simulink model "pi_OfflineRL_H2DF_2023a"  (R2023a)
settings: Solver=FixedStepAuto  StartTime=0.0  StopTime=inf  FixedStep=0.001  RelTol=1e-3  EnableMultiTasking=on
values from neighbouring files (symbols this model uses):
  C2C_NMPC = init_C2C_NMPC_H2DF(C2C_NMPC.expdata)    [init_pi_OfflineRL_H2DF_2023a.m]
  LowerLimit = ([0.17e-3;350;-2;2e-3] - C2C_NMPC.Normalization.controls.mean)./(C2C_NMPC.Normalization.controls.std)    [init_pi_OfflineRL_H2DF_2023a.m]
  UpperLimit = ([0.5e-3;900;10;5.5e-3] - C2C_NMPC.Normalization.controls.mean)./(C2C_NMPC.Normalization.controls.std)    [init_pi_OfflineRL_H2DF_2023a.m]
undefined symbols (not defined in the file or in its folder): DiscIntNeverNeededParam
libraries: deeplib x9, rllib x3, raspberrypiNetworklib x1
(part 1 of 4)
settings Model: VariantConfigurationObject=C2C  SimulationMode=external  ExtModeTrigDuration=2  Creator=maxim  LastModifiedBy=labadmin
settings SolverCC: PositivePriorityOrder=on
settings DataIOCC: LimitDataPoints=on  MaxDataPoints=10000  SaveOutput=off
settings OptimizationCC: EnhancedBackFolding=on  PassReuseOutputArgsAs=Individual arguments  ZeroExternalMemoryAtStartup=off  ZeroInternalMemoryAtStartup=off  MaxStackSize=64  OptimizeBlockOrder=speed  DifferentSizesBufferReuse=on  OptimizationCustomize=off  EfficientTunableParamExpr=on
settings DebuggingCC: ParameterPrecisionLossMsg=none  ParameterTunabilityLossMsg=error
settings HardwareCC: ProdBitPerPointer=32  ProdBitPerSizeT=32  ProdBitPerPtrDiffT=32  ProdLargestAtomicInteger=Long  ProdLargestAtomicFloat=Double  ProdWordSize=32  ProdLongLongMode=on  ProdHWDeviceType=ARM Compatible->ARM Cortex
settings RTWCC: Description=Embedded Coder  SystemTargetFile=ert.tlc  HardwareBoard=Raspberry Pi  TemplateMakefile=ert_default_tmf  RTWUseSimCustomCode=on  Toolchain=GNU GCC Embedded Linux  BuildConfiguration=Faster Runs
settings CodeAppCC: ForceParamTrailComments=on  IgnoreCustomStorageClasses=off  OperatorAnnotations=on  SimulinkDataObjDesc=on  SFDataObjDesc=on  InsertBlockDesc=on
settings ERTTargetCC: SupportContinuousTime=on  SupportNonInlinedSFcns=on  SupportVariableSizeSignals=on  ExtMode=on  ExtModeStaticAlloc=on  ExtModeMaxTrigDuration=1000  ExtModeMexArgs='192.168.140.200' 1 17725

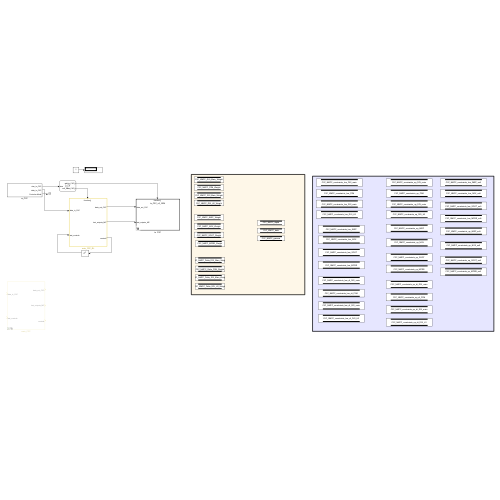
[thumbnail: Simulink's stored preview of the top-level diagram]
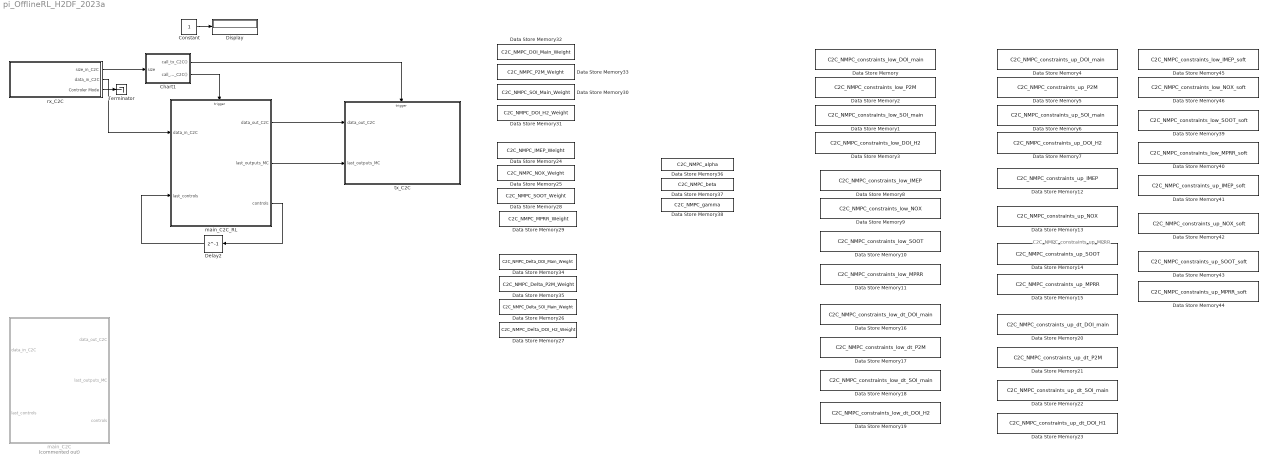
== system pi_OfflineRL_H2DF_2023a ==
  note: C2C_NMPC_constraints_up_MPRR
  Chart1 : Stateflow chart  TreatAsAtomicUnit=on
  Constant : Constant
  Data Store Memory : DataStoreMemory  DataStoreName=C2C_NMPC_constraints_low_DOI_main  WriteAfterWriteMsg=warning  ShowAdditionalParam=off
  Data Store Memory1 : DataStoreMemory  DataStoreName=C2C_NMPC_constraints_low_SOI_main  WriteAfterWriteMsg=warning  ShowAdditionalParam=off
  Data Store Memory10 : DataStoreMemory  DataStoreName=C2C_NMPC_constraints_low_SOOT  WriteAfterWriteMsg=warning  ShowAdditionalParam=off
  Data Store Memory11 : DataStoreMemory  DataStoreName=C2C_NMPC_constraints_low_MPRR  WriteAfterWriteMsg=warning  ShowAdditionalParam=off
  Data Store Memory12 : DataStoreMemory  DataStoreName=C2C_NMPC_constraints_up_IMEP  WriteAfterWriteMsg=warning  ShowAdditionalParam=off
  Data Store Memory13 : DataStoreMemory  DataStoreName=C2C_NMPC_constraints_up_NOX  WriteAfterWriteMsg=warning  ShowAdditionalParam=off
  Data Store Memory14 : DataStoreMemory  DataStoreName=C2C_NMPC_constraints_up_SOOT  WriteAfterWriteMsg=warning  ShowAdditionalParam=off
  Data Store Memory15 : DataStoreMemory  DataStoreName=C2C_NMPC_constraints_up_MPRR  WriteAfterWriteMsg=warning  ShowAdditionalParam=off
  Data Store Memory16 : DataStoreMemory  DataStoreName=C2C_NMPC_constraints_low_dt_DOI_main  WriteAfterWriteMsg=warning  ShowAdditionalParam=off
  Data Store Memory17 : DataStoreMemory  DataStoreName=C2C_NMPC_constraints_low_dt_P2M  WriteAfterWriteMsg=warning  ShowAdditionalParam=off
  Data Store Memory18 : DataStoreMemory  DataStoreName=C2C_NMPC_constraints_low_dt_SOI_main  WriteAfterWriteMsg=warning  ShowAdditionalParam=off
  Data Store Memory19 : DataStoreMemory  DataStoreName=C2C_NMPC_constraints_low_dt_DOI_H2  WriteAfterWriteMsg=warning  ShowAdditionalParam=off
  Data Store Memory2 : DataStoreMemory  DataStoreName=C2C_NMPC_constraints_low_P2M  WriteAfterWriteMsg=warning  ShowAdditionalParam=off
  Data Store Memory20 : DataStoreMemory  DataStoreName=C2C_NMPC_constraints_up_dt_DOI_main  WriteAfterWriteMsg=warning  ShowAdditionalParam=off
  Data Store Memory21 : DataStoreMemory  DataStoreName=C2C_NMPC_constraints_up_dt_P2M  WriteAfterWriteMsg=warning  ShowAdditionalParam=off
  Data Store Memory22 : DataStoreMemory  DataStoreName=C2C_NMPC_constraints_up_dt_SOI_main  WriteAfterWriteMsg=warning  ShowAdditionalParam=off
  Data Store Memory23 : DataStoreMemory  DataStoreName=C2C_NMPC_constraints_up_dt_DOI_H1  WriteAfterWriteMsg=warning  ShowAdditionalParam=off
  Data Store Memory24 : DataStoreMemory  DataStoreName=C2C_NMPC_IMEP_Weight  WriteAfterWriteMsg=warning  ShowAdditionalParam=off
  Data Store Memory25 : DataStoreMemory  DataStoreName=C2C_NMPC_NOX_Weight  WriteAfterWriteMsg=warning  ShowAdditionalParam=off
  Data Store Memory26 : DataStoreMemory  DataStoreName=C2C_NMPC_Delta_SOI_Main_Weight  WriteAfterWriteMsg=warning  ShowAdditionalParam=off
  Data Store Memory27 : DataStoreMemory  DataStoreName=C2C_NMPC_Delta_DOI_H2_Weight  WriteAfterWriteMsg=warning  ShowAdditionalParam=off
  Data Store Memory28 : DataStoreMemory  DataStoreName=C2C_NMPC_SOOT_Weight  WriteAfterWriteMsg=warning  ShowAdditionalParam=off
  Data Store Memory29 : DataStoreMemory  DataStoreName=C2C_NMPC_MPRR_Weight  WriteAfterWriteMsg=warning  ShowAdditionalParam=off
  Data Store Memory3 : DataStoreMemory  DataStoreName=C2C_NMPC_constraints_low_DOI_H2  WriteAfterWriteMsg=warning  ShowAdditionalParam=off
  Data Store Memory30 : DataStoreMemory  DataStoreName=C2C_NMPC_SOI_Main_Weight  WriteAfterWriteMsg=warning  ShowAdditionalParam=off
  Data Store Memory31 : DataStoreMemory  DataStoreName=C2C_NMPC_DOI_H2_Weight  WriteAfterWriteMsg=warning  ShowAdditionalParam=off
  Data Store Memory32 : DataStoreMemory  DataStoreName=C2C_NMPC_DOI_Main_Weight  WriteAfterWriteMsg=warning  ShowAdditionalParam=off
  Data Store Memory33 : DataStoreMemory  DataStoreName=C2C_NMPC_P2M_Weight  WriteAfterWriteMsg=warning  ShowAdditionalParam=off
  Data Store Memory34 : DataStoreMemory  DataStoreName=C2C_NMPC_Delta_DOI_Main_Weight  WriteAfterWriteMsg=warning  ShowAdditionalParam=off
  Data Store Memory35 : DataStoreMemory  DataStoreName=C2C_NMPC_Delta_P2M_Weight  WriteAfterWriteMsg=warning  ShowAdditionalParam=off
  Data Store Memory36 : DataStoreMemory  DataStoreName=C2C_NMPC_alpha  WriteAfterWriteMsg=warning  ShowAdditionalParam=off
  Data Store Memory37 : DataStoreMemory  DataStoreName=C2C_NMPC_beta  WriteAfterWriteMsg=warning  ShowAdditionalParam=off
  Data Store Memory38 : DataStoreMemory  DataStoreName=C2C_NMPC_gamma  WriteAfterWriteMsg=warning  ShowAdditionalParam=off
  Data Store Memory39 : DataStoreMemory  DataStoreName=C2C_NMPC_constraints_low_SOOT_soft  WriteAfterWriteMsg=warning  ShowAdditionalParam=off
  Data Store Memory4 : DataStoreMemory  DataStoreName=C2C_NMPC_constraints_up_DOI_main  WriteAfterWriteMsg=warning  ShowAdditionalParam=off
  Data Store Memory40 : DataStoreMemory  DataStoreName=C2C_NMPC_constraints_low_MPRR_soft  WriteAfterWriteMsg=warning  ShowAdditionalParam=off
  Data Store Memory41 : DataStoreMemory  DataStoreName=C2C_NMPC_constraints_up_IMEP_soft  WriteAfterWriteMsg=warning  ShowAdditionalParam=off
  Data Store Memory42 : DataStoreMemory  DataStoreName=C2C_NMPC_constraints_up_NOX_soft  WriteAfterWriteMsg=warning  ShowAdditionalParam=off
  Data Store Memory43 : DataStoreMemory  DataStoreName=C2C_NMPC_constraints_up_SOOT_soft  WriteAfterWriteMsg=warning  ShowAdditionalParam=off
  Data Store Memory44 : DataStoreMemory  DataStoreName=C2C_NMPC_constraints_up_MPRR_soft  WriteAfterWriteMsg=warning  ShowAdditionalParam=off
  Data Store Memory45 : DataStoreMemory  DataStoreName=C2C_NMPC_constraints_low_IMEP_soft  WriteAfterWriteMsg=warning  ShowAdditionalParam=off
  Data Store Memory46 : DataStoreMemory  DataStoreName=C2C_NMPC_constraints_low_NOX_soft  WriteAfterWriteMsg=warning  ShowAdditionalParam=off
  Data Store Memory5 : DataStoreMemory  DataStoreName=C2C_NMPC_constraints_up_P2M  WriteAfterWriteMsg=warning  ShowAdditionalParam=off
  Data Store Memory6 : DataStoreMemory  DataStoreName=C2C_NMPC_constraints_up_SOI_main  WriteAfterWriteMsg=warning  ShowAdditionalParam=off
  Data Store Memory7 : DataStoreMemory  DataStoreName=C2C_NMPC_constraints_up_DOI_H2  WriteAfterWriteMsg=warning  ShowAdditionalParam=off
  Data Store Memory8 : DataStoreMemory  DataStoreName=C2C_NMPC_constraints_low_IMEP  WriteAfterWriteMsg=warning  ShowAdditionalParam=off
  Data Store Memory9 : DataStoreMemory  DataStoreName=C2C_NMPC_constraints_low_NOX  WriteAfterWriteMsg=warning  ShowAdditionalParam=off
  Delay2 : Delay  DelayLength=1  InitialCondition=C2C_NMPC.x0([(C2C_NMPC.Dims.n_LSTM_states + 1):(C2C_NMPC.Dims.n_LSTM_states + C2C_NMPC.Dims.n_controls)])
  Display : Display
  Terminator : Terminator
  main_C2C : Subsystem  Commented=on  Variant=on  VariantControlMode=label  VariantControl=main_C2C_n3  LabelModeActiveChoice=main_C2C_RL
  main_C2C_RL : Subsystem  VariantControl=main_C2C_RL
  rx_C2C : Subsystem
  tx_C2C : Subsystem  Variant=on  VariantControlMode=label  VariantControl=Choice  LabelModeActiveChoice=tx_C2C_n3_GRU
  wires:
  rx_C2C/1(size_in_C2C) -> Chart1/1(size)
  Chart1/1(call_tx_C2C()) -> tx_C2C/Trigger
  rx_C2C/2(data_in_C2C) -> main_C2C_RL/1(data_in_C2C)
  Delay2/1 -> main_C2C_RL/2(last_controls)
  main_C2C_RL/1(data_out_C2C) -> tx_C2C/1(data_out_C2C)
  main_C2C_RL/3(controls) -> Delay2/1
  main_C2C_RL/2(last_outputs_MC) -> tx_C2C/2(last_outputs_MC)
  Constant/1 -> Display/1
  rx_C2C/3(Controler Mode) -> Terminator/1
  Chart1/2(call_main_C2C()) -> main_C2C_RL/Trigger

== system pi_OfflineRL_H2DF_2023a/main_C2C ==
  note: 192.168.140.200
  data_in_C2C : Inport
  last_controls : Inport  Port=2
  main_C2C_RL : Subsystem  VariantControl=main_C2C_RL
  data_out_C2C : Outport
  last_outputs_MC : Outport  Port=2
  controls : Outport  Port=3

== system pi_OfflineRL_H2DF_2023a/main_C2C_RL ==
  data_in_C2C : Inport
  last_controls : Inport  Port=2
  function : TriggerPort  TriggerType=function-call  VariantControl=(inherit)
  IC : InitialCondition  Value=C2C_NMPC.x0([(C2C_NMPC.Dims.n_LSTM_states + 1):(C2C_NMPC.Dims.n_LSTM_states + C2C_NMPC.Dims.n_controls)])
  RL_Controller : Subsystem  VariantControl=C2C_NMPC_n3
  post_processing : Subsystem
  pre_processing1 : Subsystem
  data_out_C2C : Outport
  last_outputs_MC : Outport  Port=2
  controls : Outport  Port=3
  wires:
  post_processing/1(data_C2C_out) -> data_out_C2C/1
  pre_processing1/2(counter_C2C) -> [counter_C2C]
  [counter_C2C] -> post_processing/5(counter)
  last_controls/1 -> [last_controls]
  RL_Controller/1(status_C2C) -> post_processing/3(controller_status)
  [last_outputs_MC] -> post_processing/4(last_outputs_MC)
  [last_outputs_MC] -> last_outputs_MC/1
  pre_processing1/3(last_outputs_MC) -> RL_Controller/2(last_outputs), [last_outputs_MC]
  data_in_C2C/1 -> pre_processing1/1(data_in_C2C)
  pre_processing1/1(reference_C2C) -> post_processing/1(reference), RL_Controller/1(reference_C2C)
  IC/1 -> controls/1, post_processing/2(controls)
  RL_Controller/3(LSTM_states) -> post_processing/6(LSTM_States)
  RL_Controller/2(controls) -> IC/1

== system pi_OfflineRL_H2DF_2023a/rx_C2C ==
  Data Type Conversion : DataTypeConversion  OutDataTypeStr=double  SaturateOnIntegerOverflow=off  RndMeth=Floor
  Receive : Subsystem
  Subsystem1 : Subsystem  Commented=on
  Subsystem4 : Subsystem  Commented=on
  UDP Receive1 : raspberrypiNetworklib/UDP Receive  localURL='0.0.0.0'  localPort=42785  remoteURL='0.0.0.0'  remotePort=-1  recvBufferSize=8192  signalDatatype=uint32  dims=56  isVarSize=off  showBlockingTime=off  blockingTime=0  sampletime=0.001  blockPlatform=Raspberry Pi
  size_in_C2C : Outport
  data_in_C2C : Outport  Port=2
  Controler Mode : Outport  Port=3
  wires:
  UDP Receive1/2 -> size_in_C2C/1
  UDP Receive1/1 -> Data Type Conversion/1
  Receive/1(udp_outputs) -> data_in_C2C/1
  Data Type Conversion/1 -> Receive/1(udp_data_in)
  Receive/2(controller_mode) -> Controler Mode/1

== system pi_OfflineRL_H2DF_2023a/tx_C2C ==
  data_out_C2C : Inport
  last_outputs_MC : Inport  Port=2
  function : TriggerPort  TriggerType=function-call  VariantControl=(inherit)
  tx_C2C_n3 : Subsystem  VariantControl=tx_C2C_n3
  tx_C2C_n3_GRU : Subsystem  VariantControl=tx_C2C_n3_GRU

== system pi_OfflineRL_H2DF_2023a/main_C2C/main_C2C_RL ==
  data_in_C2C : Inport
  last_controls : Inport  Port=2
  IC : InitialCondition  Value=C2C_NMPC.x0([(C2C_NMPC.Dims.n_LSTM_states + 1):(C2C_NMPC.Dims.n_LSTM_states + C2C_NMPC.Dims.n_controls)])
  RL_Controller : Subsystem  VariantControl=C2C_NMPC_n3
  post_processing : Subsystem
  pre_processing1 : Subsystem
  data_out_C2C : Outport
  last_outputs_MC : Outport  Port=2
  controls : Outport  Port=3
  wires:
  post_processing/1(data_C2C_out) -> data_out_C2C/1
  pre_processing1/2(counter_C2C) -> [counter_C2C]
  [counter_C2C] -> post_processing/5(counter)
  last_controls/1 -> [last_controls]
  RL_Controller/1(status_C2C) -> post_processing/3(controller_status)
  [last_outputs_MC] -> post_processing/4(last_outputs_MC)
  [last_outputs_MC] -> last_outputs_MC/1
  pre_processing1/3(last_outputs_MC) -> RL_Controller/2(last_outputs), [last_outputs_MC]
  data_in_C2C/1 -> pre_processing1/1(data_in_C2C)
  pre_processing1/1(reference_C2C) -> post_processing/1(reference), RL_Controller/1(reference_C2C)
  IC/1 -> controls/1, post_processing/2(controls)
  RL_Controller/3(LSTM_states) -> post_processing/6(LSTM_States)
  RL_Controller/2(controls) -> IC/1

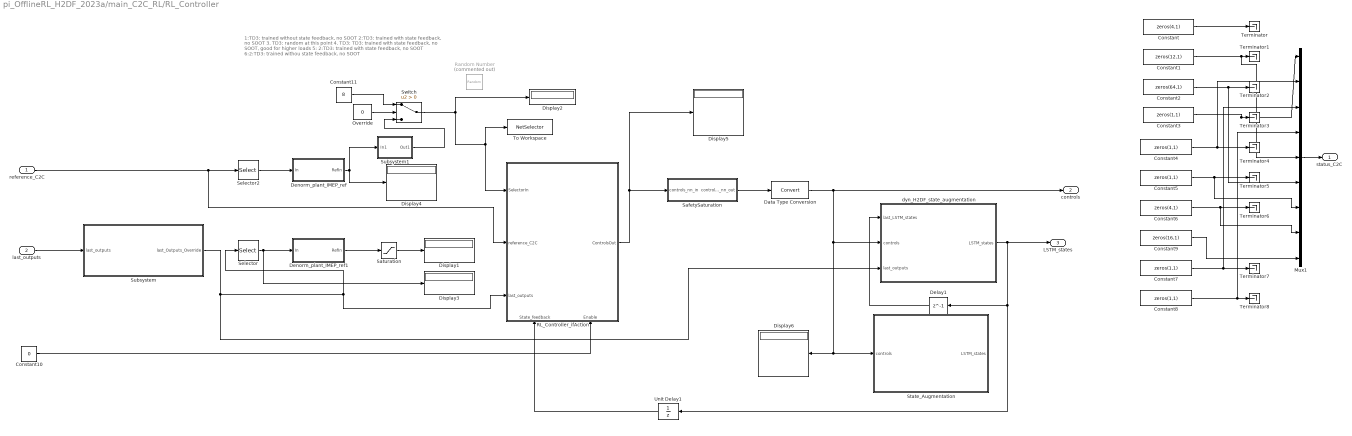
== system pi_OfflineRL_H2DF_2023a/main_C2C_RL/RL_Controller ==
  note: 1:TD3: trained without state feedback, no SOOT
      | 2:TD3: trained with state feedback, no SOOT
      | 3. TD3: random at this point
      | 4. TD3: TD3: trained with state feedback, no SOOT, good for higher loads
      | 5: 2:TD3: trained with state feedback, no SOOT
      | 6:2:TD3: trained withou state feedback, no SOOT
  reference_C2C : Inport
  last_outputs : Inport  Port=2
  Constant : Constant  Value=zeros(4,1)
  Constant1 : Constant  Value=zeros(12,1)
  Constant10 : Constant  Value=0
  Constant11 : Constant  Value=8
  Constant2 : Constant  Value=zeros(64,1)
  Constant{3..5,7..8} (5 alike) : Constant  Value=zeros(1,1)
  Constant6 : Constant  Value=zeros(4,1)
  Constant9 : Constant  Value=zeros(16,1)
  Data Type Conversion : DataTypeConversion  SaturateOnIntegerOverflow=off  RndMeth=Floor
  Delay1 : Delay  DelayLength=1  InitialCondition=C2C_NMPC.x0(1:C2C_NMPC.Dims.n_LSTM_states)
  Denorm_plant_IMEP_ref : Subsystem
  Denorm_plant_IMEP_ref1 : Subsystem
  Display{1..6} (6 alike) : Display
  Mux1 : Mux  Inputs=9
  Override : Constant  Value=0
  RL_Controller_ifAction : Subsystem  TreatAsAtomicUnit=on  PartitionName=part1
      settings: PortSchema="{\"entries\":[{\"content\":{\"sides\":[{\"content\":{\"connectorIds\":[\"In1\",\"In2\",\"In3\"]},\"type\":\"ConnectorPlacement.EquallySpacedRectSide\",\"uuid\":\"a8c8a062-4d7f-4cb6-97fb-36445aa99a41\"},{\"content\":{\"connectorIds\":[\"Out1\"],\"side\":\"RIGHT\"},\"type\":\"ConnectorPlacement.EquallySpacedRectSide\",\"uuid\":\"6b7bd18d-d80d-4e99-9545-a79fc8c73da4\"},{\"content\":{\"side\":\"TOP\"},\"type\":\"ConnectorPlacement.EquallySpacedRectSide\",\"uuid\":\"fed7c1b0-30f7-49dc-b931-1771d032fe96\"},{\"content\":{\"connectorIds\":[\"In4\",\"In5\"],\"side\":\"BOTTOM\"},\"type\":\"ConnectorPlacement.EquallySpacedRectSide\",\"uuid\":\"e54c4c0f-d141-48ae-a9a4-98bc154936a6\"}]},\"type\":\"ConnectorPlacement.EquallySpacedConnector\",\"uuid\":\"17160fdf-37bf-457c-841e-5f362c3aef18\"}],\"packageUris\":[\"http://schema.mathworks.com/mf0/Connector/R2020b\"],\"version\":\"1.0\"}"
  Random Number : RandomNumber  Commented=on
  SafetySaturation : Subsystem
  Saturation : Saturate  UpperLimit=8.5e5  LowerLimit=3e5
  Selector : Selector  InputPortWidth=4  IndexOptions=Index vector (dialog)  Indices=[1]  OutputSizes=1
  Selector2 : Selector  IndexOptions=Index vector (dialog)  Indices=5  OutputSizes=1
  State_Augmentation : Subsystem
  Subsystem : Subsystem
  Subsystem1 : Subsystem
  Switch : Switch  Criteria=u2 > Threshold  SaturateOnIntegerOverflow=off  InputSameDT=off
  Terminator{,1..8} (9 alike) : Terminator
  To Workspace : ToWorkspace  VariableName=NetSelector  SampleTime=-1
      settings: Save2DSignal=2-D array (concatenate along first dimension)
  Unit Delay1 : UnitDelay  SampleTime=-1  HasFrameUpgradeWarning=on
  dyn_H2DF_state_augmentation : Subsystem
  status_C2C : Outport
  controls : Outport  Port=2
  LSTM_states : Outport  Port=3
  wires:
  Constant4/1 -> Mux1/2, Terminator4/1
  Mux1/1 -> status_C2C/1
  Constant8/1 -> Terminator8/1, Mux1/4
  Constant7/1 -> Terminator7/1, Mux1/3
  Constant6/1 -> Terminator6/1, Mux1/8
  Constant5/1 -> Terminator5/1, Mux1/7
  Constant9/1 -> Mux1/9
  Constant3/1 -> Mux1/1, Terminator3/1
  Constant2/1 -> Terminator2/1, Mux1/6
  Constant1/1 -> Terminator1/1, Mux1/5
  Constant/1 -> Terminator/1
  Selector2/1 -> Denorm_plant_IMEP_ref/1(In)
  Saturation/1 -> Display1/1
  reference_C2C/1 -> RL_Controller_ifAction/2(reference_C2C), Selector2/1
  Selector/1 -> Denorm_plant_IMEP_ref1/1(In), Display3/1
  Denorm_plant_IMEP_ref/1(RefIn) -> Subsystem1/1(In1), Display4/1
  Denorm_plant_IMEP_ref1/1(RefIn) -> Saturation/1
  last_outputs/1 -> Subsystem/1(last_outputs)
  Switch/1 -> Display2/1, RL_Controller_ifAction/1(SelectorIn), To Workspace/1
  SafetySaturation/1(controls_nn_out) -> Data Type Conversion/1
  RL_Controller_ifAction/1(ControlsOut) -> Display5/1, SafetySaturation/1(controls_nn_in)
  Data Type Conversion/1 -> State_Augmentation/1(controls), Display6/1, dyn_H2DF_state_augmentation/2(controls), controls/1
  Constant10/1 -> RL_Controller_ifAction/5(Enable)
  Subsystem/1(last_Outputs_Override) -> dyn_H2DF_state_augmentation/3(last_outputs), RL_Controller_ifAction/3(last_outputs), Selector/1
  dyn_H2DF_state_augmentation/1(LSTM_states) -> LSTM_states/1, Unit Delay1/1, Delay1/1
  Delay1/1 -> dyn_H2DF_state_augmentation/1(last_LSTM_states)
  Unit Delay1/1 -> RL_Controller_ifAction/4(State_feedback)
  Override/1 -> Switch/2
  Subsystem1/1(Out1) -> Switch/3
  Constant11/1 -> Switch/1

== system pi_OfflineRL_H2DF_2023a/main_C2C_RL/post_processing ==
  reference : Inport
  controls : Inport  Port=2
  controller_status : Inport  Port=3
  last_outputs_MC : Inport  Port=4
  counter : Inport  Port=5
  LSTM_States : Inport  Port=6
  " denormalizing reference" : Subsystem
  Demux1 : Demux
  Demux2 : Demux
  Demux3 : Demux
  Display : Display  Commented=on
  Display1 : Display
  Mux{1,8..11} (5 alike) : Mux  Inputs=2
  Mux4 : Mux
  Mux5 : Mux  Inputs=6
  Mux6 : Mux
  Selector5 : Selector  IndexOptions=Index vector (dialog)  Indices=[(C2C_NMPC.Dims.n_controls + 1 ):(C2C_NMPC.Dims.n_cost - C2C_NMPC.Dims.n_controls)]  OutputSizes=1
  Subsystem : Subsystem  Commented=on
  Subsystem1 : Subsystem
  denormalizing physical controls and outputs : Subsystem
  data_C2C_out : Outport
  wires:
  Demux3/1 -> " denormalizing reference"/1(IMEP_norm)
  Demux3/2 -> " denormalizing reference"/2(NOX_norm)
  Demux3/4 -> " denormalizing reference"/4(MPRR_norm)
  Demux3/3 -> " denormalizing reference"/3(soot_norm)
  reference/1 -> Selector5/1
  Selector5/1 -> Demux3/1
  controls/1 -> Demux2/1
  Demux1/1 -> denormalizing physical controls and outputs/1(IMEP_norm)
  Demux1/2 -> denormalizing physical controls and outputs/2(NOX_norm)
  Demux1/3 -> denormalizing physical controls and outputs/3(soot_norm)
  Demux1/4 -> denormalizing physical controls and outputs/4(MPRR_norm)
  Demux2/1 -> denormalizing physical controls and outputs/5(DOI_main_norm)
  Demux2/2 -> denormalizing physical controls and outputs/6(SOI_pre_norm)
  Demux2/3 -> denormalizing physical controls and outputs/7(SOI_main_norm)
  denormalizing physical controls and outputs/5(DOI_main) -> Mux6/1
  denormalizing physical controls and outputs/6(SOI_pre) -> Mux6/2
  denormalizing physical controls and outputs/7(SOI_main) -> Mux6/3
  " denormalizing reference"/1(IMEP) -> Mux11/1
  " denormalizing reference"/2(NOX) -> Mux9/1
  " denormalizing reference"/3(soot) -> Mux8/1
  " denormalizing reference"/4(MPRR) -> Mux10/1
  controller_status/1 -> Mux5/4, Subsystem1/1(controller_ status), Subsystem/1(controller_ status)
  Mux5/1 -> data_C2C_out/1
  Mux8/1 -> Mux4/3
  Mux10/1 -> Mux4/4
  denormalizing physical controls and outputs/1(IMEP) -> Mux11/2
  denormalizing physical controls and outputs/2(NOX) -> Mux9/2
  denormalizing physical controls and outputs/3(soot) -> Mux8/2
  denormalizing physical controls and outputs/4(MPRR) -> Mux10/2
  Mux4/1 -> Mux5/2
  counter/1 -> Mux5/3
  Mux6/1 -> Display/1, Mux5/1
  Demux2/4 -> denormalizing physical controls and outputs/8(DOI_H2_norm)
  denormalizing physical controls and outputs/8(DOI_H2) -> Mux6/4
  Mux9/1 -> Mux4/2
  last_outputs_MC/1 -> Subsystem1/2(Last_Output_MC), Demux1/1
  Subsystem1/1(Out1) -> Mux5/6
  Mux11/1 -> Display1/1, Mux4/1
  LSTM_States/1 -> Mux1/2, Mux1/1
  Mux1/1 -> Mux5/5

== system pi_OfflineRL_H2DF_2023a/main_C2C_RL/pre_processing1 ==
  data_in_C2C : Inport
  Selector : Selector  IndexOptions=Index vector (dialog)  Indices=[6]  OutputSizes=1
  normalize_last_outputs_MC : Subsystem
  normalize_reference_C2C : Subsystem
  reference_C2C : Outport  VectorParamsAs1DForOutWhenUnconnected=off
  counter_C2C : Outport  Port=2  VectorParamsAs1DForOutWhenUnconnected=off
  last_outputs_MC : Outport  Port=3  VectorParamsAs1DForOutWhenUnconnected=off
  wires:
  normalize_reference_C2C/1(reference_C2C) -> reference_C2C/1
  data_in_C2C/1 -> Selector/1, normalize_last_outputs_MC/1(data_in), normalize_reference_C2C/1(data_in)
  normalize_last_outputs_MC/1(last_outputs_MC) -> last_outputs_MC/1
  Selector/1 -> counter_C2C/1

== system pi_OfflineRL_H2DF_2023a/rx_C2C/Receive ==
  note: block for horizon of 3 from engine
  note: block for horizon of 1 from engine
  udp_data_in : Inport
  conversion_n1 : Subsystem  Commented=on
  conversion_n3 : Subsystem
  udp_outputs : Outport
  controller_mode : Outport  Port=2
  wires:
  udp_data_in/1 -> conversion_n3/1(udp_data_in)
  conversion_n3/1(udp_outputs) -> udp_outputs/1
  conversion_n3/2(controller_mode) -> controller_mode/1

== system pi_OfflineRL_H2DF_2023a/rx_C2C/Subsystem1 ==
  Data Store Write : DataStoreWrite  DataStoreName=C2C_NMPC_IMEP_Weight  IndexOptions=Index vector (dialog)  Indices=1  OutputSizes=1
  Data Store Write1 : DataStoreWrite  DataStoreName=C2C_NMPC_NOX_Weight  IndexOptions=Index vector (dialog)  Indices=1  OutputSizes=1
  Data Store Write10 : DataStoreWrite  DataStoreName=C2C_NMPC_Delta_SOI_Main_Weight  IndexOptions=Index vector (dialog)  Indices=1  OutputSizes=1
  Data Store Write11 : DataStoreWrite  DataStoreName=C2C_NMPC_Delta_DOI_H2_Weight  IndexOptions=Index vector (dialog)  Indices=1  OutputSizes=1
  Data Store Write2 : DataStoreWrite  DataStoreName=C2C_NMPC_SOOT_Weight  IndexOptions=Index vector (dialog)  Indices=1  OutputSizes=1
  Data Store Write3 : DataStoreWrite  DataStoreName=C2C_NMPC_MPRR_Weight  IndexOptions=Index vector (dialog)  Indices=1  OutputSizes=1
  Data Store Write4 : DataStoreWrite  DataStoreName=C2C_NMPC_DOI_Main_Weight  IndexOptions=Index vector (dialog)  Indices=1  OutputSizes=1
  Data Store Write5 : DataStoreWrite  DataStoreName=C2C_NMPC_P2M_Weight  IndexOptions=Index vector (dialog)  Indices=1  OutputSizes=1
  Data Store Write6 : DataStoreWrite  DataStoreName=C2C_NMPC_SOI_Main_Weight  IndexOptions=Index vector (dialog)  Indices=1  OutputSizes=1
  Data Store Write7 : DataStoreWrite  DataStoreName=C2C_NMPC_DOI_H2_Weight  IndexOptions=Index vector (dialog)  Indices=1  OutputSizes=1
  Data Store Write8 : DataStoreWrite  DataStoreName=C2C_NMPC_Delta_DOI_Main_Weight  IndexOptions=Index vector (dialog)  Indices=1  OutputSizes=1
  Data Store Write9 : DataStoreWrite  DataStoreName=C2C_NMPC_Delta_P2M_Weight  IndexOptions=Index vector (dialog)  Indices=1  OutputSizes=1
  weight_IMEP : Constant  Value=8
  weight_Nox1 : Constant  Value=0
  weight_dt_u_1 : Constant
  weight_dt_u_2 : Constant
  weight_dt_u_3 : Constant
  weight_dt_u_4 : Constant  Value=10
  weight_mprr1 : Constant  Value=0.5
  weight_soot : Constant  Value=0
  weight_u_1 : Constant
  weight_u_2 : Constant  Value=0
  weight_u_3 : Constant  Value=0
  weight_u_4 : Constant  Value=0.1
  wires:
  weight_soot/1 -> Data Store Write2/1
  weight_dt_u_4/1 -> Data Store Write11/1
  weight_dt_u_1/1 -> Data Store Write8/1
  weight_mprr1/1 -> Data Store Write3/1
  weight_dt_u_3/1 -> Data Store Write10/1
  weight_dt_u_2/1 -> Data Store Write9/1
  weight_Nox1/1 -> Data Store Write1/1
  weight_u_3/1 -> Data Store Write6/1
  weight_u_4/1 -> Data Store Write7/1
  weight_u_1/1 -> Data Store Write4/1
  weight_IMEP/1 -> Data Store Write/1
  weight_u_2/1 -> Data Store Write5/1

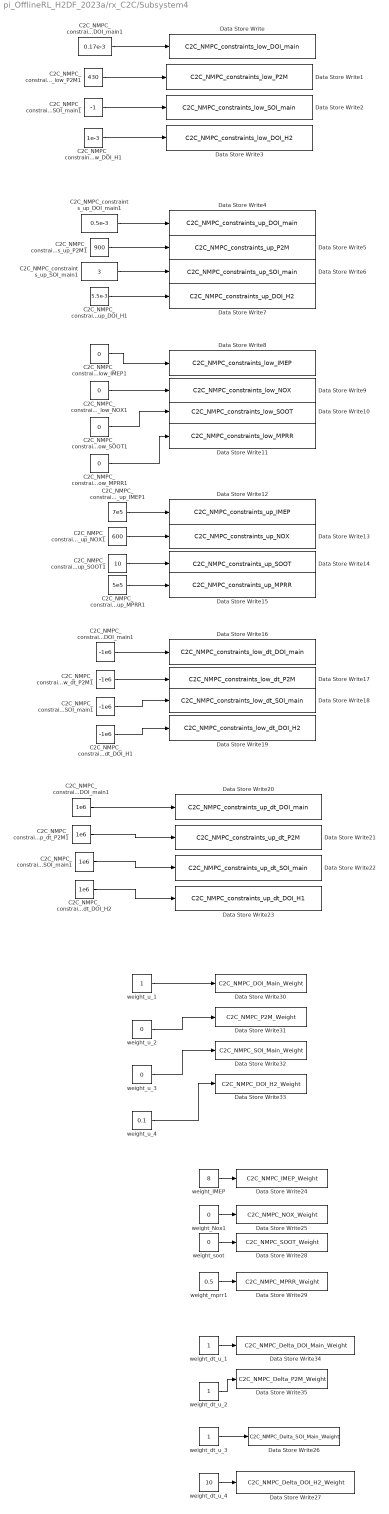
== system pi_OfflineRL_H2DF_2023a/rx_C2C/Subsystem4 ==
  C2C_NMPC_constraints_low_DOI_H1 : Constant  Value=1e-3
  C2C_NMPC_constraints_low_DOI_main1 : Constant  Value=0.17e-3
  C2C_NMPC_constraints_low_IMEP1 : Constant  Value=0
  C2C_NMPC_constraints_low_MPRR1 : Constant  Value=0
  C2C_NMPC_constraints_low_NOX1 : Constant  Value=0
  C2C_NMPC_constraints_low_P2M1 : Constant  Value=430
  C2C_NMPC_constraints_low_SOI_main1 : Constant  Value=-1
  C2C_NMPC_constraints_low_SOOT1 : Constant  Value=0
  C2C_NMPC_constraints_low_dt_DOI_H1 : Constant  Value=-1e6
  C2C_NMPC_constraints_low_dt_DOI_main1 : Constant  Value=-1e6
  C2C_NMPC_constraints_low_dt_P2M1 : Constant  Value=-1e6
  C2C_NMPC_constraints_low_dt_SOI_main1 : Constant  Value=-1e6
  C2C_NMPC_constraints_up_DOI_H1 : Constant  Value=5.5e-3
  C2C_NMPC_constraints_up_DOI_main1 : Constant  Value=0.5e-3
  C2C_NMPC_constraints_up_IMEP1 : Constant  Value=7e5
  C2C_NMPC_constraints_up_MPRR1 : Constant  Value=5e5
  C2C_NMPC_constraints_up_NOX1 : Constant  Value=600
  C2C_NMPC_constraints_up_P2M1 : Constant  Value=900
  C2C_NMPC_constraints_up_SOI_main1 : Constant  Value=3
  C2C_NMPC_constraints_up_SOOT1 : Constant  Value=10
  C2C_NMPC_constraints_up_dt_DOI_H2 : Constant  Value=1e6
  C2C_NMPC_constraints_up_dt_DOI_main1 : Constant  Value=1e6
  C2C_NMPC_constraints_up_dt_P2M1 : Constant  Value=1e6
  C2C_NMPC_constraints_up_dt_SOI_main1 : Constant  Value=1e6
  Data Store Write : DataStoreWrite  DataStoreName=C2C_NMPC_constraints_low_DOI_main  IndexOptions=Index vector (dialog)  Indices=1  OutputSizes=1
  Data Store Write1 : DataStoreWrite  DataStoreName=C2C_NMPC_constraints_low_P2M  IndexOptions=Index vector (dialog)  Indices=1  OutputSizes=1
  Data Store Write10 : DataStoreWrite  DataStoreName=C2C_NMPC_constraints_low_SOOT  IndexOptions=Index vector (dialog)  Indices=1  OutputSizes=1
  Data Store Write11 : DataStoreWrite  DataStoreName=C2C_NMPC_constraints_low_MPRR  IndexOptions=Index vector (dialog)  Indices=1  OutputSizes=1
  Data Store Write12 : DataStoreWrite  DataStoreName=C2C_NMPC_constraints_up_IMEP  IndexOptions=Index vector (dialog)  Indices=1  OutputSizes=1
  Data Store Write13 : DataStoreWrite  DataStoreName=C2C_NMPC_constraints_up_NOX  IndexOptions=Index vector (dialog)  Indices=1  OutputSizes=1
  Data Store Write14 : DataStoreWrite  DataStoreName=C2C_NMPC_constraints_up_SOOT  IndexOptions=Index vector (dialog)  Indices=1  OutputSizes=1
  Data Store Write15 : DataStoreWrite  DataStoreName=C2C_NMPC_constraints_up_MPRR  IndexOptions=Index vector (dialog)  Indices=1  OutputSizes=1
  Data Store Write16 : DataStoreWrite  DataStoreName=C2C_NMPC_constraints_low_dt_DOI_main  IndexOptions=Index vector (dialog)  Indices=1  OutputSizes=1
  Data Store Write17 : DataStoreWrite  DataStoreName=C2C_NMPC_constraints_low_dt_P2M  IndexOptions=Index vector (dialog)  Indices=1  OutputSizes=1
  Data Store Write18 : DataStoreWrite  DataStoreName=C2C_NMPC_constraints_low_dt_SOI_main  IndexOptions=Index vector (dialog)  Indices=1  OutputSizes=1
  Data Store Write19 : DataStoreWrite  DataStoreName=C2C_NMPC_constraints_low_dt_DOI_H2  IndexOptions=Index vector (dialog)  Indices=1  OutputSizes=1
  Data Store Write2 : DataStoreWrite  DataStoreName=C2C_NMPC_constraints_low_SOI_main  IndexOptions=Index vector (dialog)  Indices=1  OutputSizes=1
  Data Store Write20 : DataStoreWrite  DataStoreName=C2C_NMPC_constraints_up_dt_DOI_main  IndexOptions=Index vector (dialog)  Indices=1  OutputSizes=1
  Data Store Write21 : DataStoreWrite  DataStoreName=C2C_NMPC_constraints_up_dt_P2M  IndexOptions=Index vector (dialog)  Indices=1  OutputSizes=1
  Data Store Write22 : DataStoreWrite  DataStoreName=C2C_NMPC_constraints_up_dt_SOI_main  IndexOptions=Index vector (dialog)  Indices=1  OutputSizes=1
  Data Store Write23 : DataStoreWrite  DataStoreName=C2C_NMPC_constraints_up_dt_DOI_H1  IndexOptions=Index vector (dialog)  Indices=1  OutputSizes=1
  Data Store Write24 : DataStoreWrite  DataStoreName=C2C_NMPC_IMEP_Weight  IndexOptions=Index vector (dialog)  Indices=1  OutputSizes=1
  Data Store Write25 : DataStoreWrite  DataStoreName=C2C_NMPC_NOX_Weight  IndexOptions=Index vector (dialog)  Indices=1  OutputSizes=1
  Data Store Write26 : DataStoreWrite  DataStoreName=C2C_NMPC_Delta_SOI_Main_Weight  IndexOptions=Index vector (dialog)  Indices=1  OutputSizes=1
  Data Store Write27 : DataStoreWrite  DataStoreName=C2C_NMPC_Delta_DOI_H2_Weight  IndexOptions=Index vector (dialog)  Indices=1  OutputSizes=1
  Data Store Write28 : DataStoreWrite  DataStoreName=C2C_NMPC_SOOT_Weight  IndexOptions=Index vector (dialog)  Indices=1  OutputSizes=1
  Data Store Write29 : DataStoreWrite  DataStoreName=C2C_NMPC_MPRR_Weight  IndexOptions=Index vector (dialog)  Indices=1  OutputSizes=1
  Data Store Write3 : DataStoreWrite  DataStoreName=C2C_NMPC_constraints_low_DOI_H2  IndexOptions=Index vector (dialog)  Indices=1  OutputSizes=1
  Data Store Write30 : DataStoreWrite  DataStoreName=C2C_NMPC_DOI_Main_Weight  IndexOptions=Index vector (dialog)  Indices=1  OutputSizes=1
  Data Store Write31 : DataStoreWrite  DataStoreName=C2C_NMPC_P2M_Weight  IndexOptions=Index vector (dialog)  Indices=1  OutputSizes=1
  Data Store Write32 : DataStoreWrite  DataStoreName=C2C_NMPC_SOI_Main_Weight  IndexOptions=Index vector (dialog)  Indices=1  OutputSizes=1
  Data Store Write33 : DataStoreWrite  DataStoreName=C2C_NMPC_DOI_H2_Weight  IndexOptions=Index vector (dialog)  Indices=1  OutputSizes=1
  Data Store Write34 : DataStoreWrite  DataStoreName=C2C_NMPC_Delta_DOI_Main_Weight  IndexOptions=Index vector (dialog)  Indices=1  OutputSizes=1
  Data Store Write35 : DataStoreWrite  DataStoreName=C2C_NMPC_Delta_P2M_Weight  IndexOptions=Index vector (dialog)  Indices=1  OutputSizes=1
  Data Store Write4 : DataStoreWrite  DataStoreName=C2C_NMPC_constraints_up_DOI_main  IndexOptions=Index vector (dialog)  Indices=1  OutputSizes=1
  Data Store Write5 : DataStoreWrite  DataStoreName=C2C_NMPC_constraints_up_P2M  IndexOptions=Index vector (dialog)  Indices=1  OutputSizes=1
  Data Store Write6 : DataStoreWrite  DataStoreName=C2C_NMPC_constraints_up_SOI_main  IndexOptions=Index vector (dialog)  Indices=1  OutputSizes=1
  Data Store Write7 : DataStoreWrite  DataStoreName=C2C_NMPC_constraints_up_DOI_H2  IndexOptions=Index vector (dialog)  Indices=1  OutputSizes=1
  Data Store Write8 : DataStoreWrite  DataStoreName=C2C_NMPC_constraints_low_IMEP  IndexOptions=Index vector (dialog)  Indices=1  OutputSizes=1
  Data Store Write9 : DataStoreWrite  DataStoreName=C2C_NMPC_constraints_low_NOX  IndexOptions=Index vector (dialog)  Indices=1  OutputSizes=1
  weight_IMEP : Constant  Value=8
  weight_Nox1 : Constant  Value=0
  weight_dt_u_1 : Constant
  weight_dt_u_2 : Constant
  weight_dt_u_3 : Constant
  weight_dt_u_4 : Constant  Value=10
  weight_mprr1 : Constant  Value=0.5
  weight_soot : Constant  Value=0
  weight_u_1 : Constant
  weight_u_2 : Constant  Value=0
  weight_u_3 : Constant  Value=0
  weight_u_4 : Constant  Value=0.1
  wires:
  C2C_NMPC_constraints_up_NOX1/1 -> Data Store Write13/1
  C2C_NMPC_constraints_up_dt_P2M1/1 -> Data Store Write21/1
  C2C_NMPC_constraints_low_dt_SOI_main1/1 -> Data Store Write18/1
  C2C_NMPC_constraints_up_dt_DOI_main1/1 -> Data Store Write20/1
  C2C_NMPC_constraints_low_dt_P2M1/1 -> Data Store Write17/1
  C2C_NMPC_constraints_up_dt_SOI_main1/1 -> Data Store Write22/1
  C2C_NMPC_constraints_up_DOI_main1/1 -> Data Store Write4/1
  C2C_NMPC_constraints_low_SOI_main1/1 -> Data Store Write2/1
  C2C_NMPC_constraints_up_P2M1/1 -> Data Store Write5/1
  C2C_NMPC_constraints_up_IMEP1/1 -> Data Store Write12/1
  C2C_NMPC_constraints_low_P2M1/1 -> Data Store Write1/1
  C2C_NMPC_constraints_up_SOOT1/1 -> Data Store Write14/1
  C2C_NMPC_constraints_up_MPRR1/1 -> Data Store Write15/1
  C2C_NMPC_constraints_low_dt_DOI_main1/1 -> Data Store Write16/1
  C2C_NMPC_constraints_low_DOI_main1/1 -> Data Store Write/1
  C2C_NMPC_constraints_low_dt_DOI_H1/1 -> Data Store Write19/1
  C2C_NMPC_constraints_low_MPRR1/1 -> Data Store Write11/1
  C2C_NMPC_constraints_low_DOI_H1/1 -> Data Store Write3/1
  C2C_NMPC_constraints_low_NOX1/1 -> Data Store Write9/1
  C2C_NMPC_constraints_low_IMEP1/1 -> Data Store Write8/1
  C2C_NMPC_constraints_up_SOI_main1/1 -> Data Store Write6/1
  C2C_NMPC_constraints_low_SOOT1/1 -> Data Store Write10/1
  C2C_NMPC_constraints_up_dt_DOI_H2/1 -> Data Store Write23/1
  C2C_NMPC_constraints_up_DOI_H1/1 -> Data Store Write7/1
  weight_dt_u_2/1 -> Data Store Write35/1
  weight_u_3/1 -> Data Store Write32/1
  weight_u_4/1 -> Data Store Write33/1
  weight_IMEP/1 -> Data Store Write24/1
  weight_u_1/1 -> Data Store Write30/1
  weight_Nox1/1 -> Data Store Write25/1
  weight_dt_u_3/1 -> Data Store Write26/1
  weight_mprr1/1 -> Data Store Write29/1
  weight_dt_u_4/1 -> Data Store Write27/1
  weight_soot/1 -> Data Store Write28/1
  weight_dt_u_1/1 -> Data Store Write34/1
  weight_u_2/1 -> Data Store Write31/1

== system pi_OfflineRL_H2DF_2023a/tx_C2C/tx_C2C_n3 ==
  data_out_C2C : Inport
  last_outputs_MC : Inport  Port=2
  function : TriggerPort  TriggerType=function-call  VariantControl=(inherit)
  Constant : Constant  Commented=on  Value=2*linspace(1,39,39)
  Data Type Conversion : DataTypeConversion  OutDataTypeStr=uint32  SaturateOnIntegerOverflow=off  RndMeth=Floor
  Selector : Selector  IndexOptions=Index vector (dialog)  Indices=[1:4,13,155:190,14:17,127:130]  OutputSizes=1
  Subsystem : Subsystem
  UDP Send1 : S-Function  AncestorBlock=raspberrypiNetworklib/UDP Send  InitFcn=|  FunctionName=sdspToNetwork  Parameters=localURL, localPortSource, localPort, remoteURL, remotePort, 8192, separateLengthPort, []  SFunctionDeploymentMode=off  EnableBusSupport=off  mask(UDP Send){remoteURL='192.168.140.159', remotePort=42784, localURL='0.0.0.0', localPortSource=Specify via dialog, localPort=42784, sampletime=-1, blockPlatform=Raspberry Pi, separateLengthPort=0}
      | realtime.internal.validateLinuxBlock(get_param(gcbh, 'blockPlatform'), gcbh);
      | realtime.internal.registerLinuxBlock(gcb);
      mask prompts: remoteURL "Remote IP address ('255.255.255.255' for broadcast):"; remotePort "Remote IP port:"; localURL "Local IP address:"; localPortSource "Local IP port source:"; localPort "Local IP port:"; blockPlatform "Block Platform"; separateLengthPort "Use a separate length port"
      mask help: Sends UDP packets to another UDP host on an Internet network. Set Remote IP address parameter to the IP address of the receiving UDP host. Set the Remote IP port parameter to the port number used by the receiving UDP host.
      mask Help: eval('realtime.helpView(get_param(gcb, ''blockPlatform''), [realtime.internal.getHelpLinkPrefix(gcb) ''libudpsend''])');
      mask TypeOptions localPortSource: Automatically determine | Specify via dialog
      mask Callback localPortSource:
      | mask_vis = get_param(gcbh, 'MaskVisibilities');
      | if strcmp(get_param(gcbh,'localPortSource'),'Specify via dialog')
      |     mask_vis{5} = 'on';
      | else
      |     mask_vis{5} = 'off';
      | end
      | set_param(gcbh, 'MaskVisibilities', mask_vis);
      | clear('mask_vis');
      mask Display:
      | %fprintf('UDP Send');
      | color('blue');
      | [data, map]=imread('ethernet2_bw.gif');pic=ind2rgb(data,map);image(pic,[0.32 0.25 0.40 0.45]);
      | platform = realtime.internal.getBlockDisplayText(gcb);
      | text(0.99, 0.9, platform, 'horizontalalignment', 'right');
  encode : MATLAB Function  Commented=on  TreatAsAtomicUnit=on
  wires:
  encode/1(serialized_data) -> ?
  data_out_C2C/1 -> Selector/1
  Data Type Conversion/1 -> UDP Send1/1
  Subsystem/1(Out1) -> Data Type Conversion/1
  Selector/1 -> Subsystem/1(In1)

== system pi_OfflineRL_H2DF_2023a/tx_C2C/tx_C2C_n3_GRU ==
  note: [1:4,13,99:134,14,15,16,17,71:74]
  data_out_C2C : Inport
  last_outputs_MC : Inport  Port=2
  function : TriggerPort  TriggerType=function-call  VariantControl=(inherit)
  Constant : Constant  Commented=on  Value=2*linspace(1,39,39)
  Data Type Conversion : DataTypeConversion  OutDataTypeStr=uint32  SaturateOnIntegerOverflow=off  RndMeth=Floor
  Selector : Selector  IndexOptions=Index vector (dialog)  Indices=[1:4,13,115:142,14,15,16,17,95:98]  OutputSizes=1
  Subsystem : Subsystem
  UDP Send1 : S-Function  AncestorBlock=raspberrypiNetworklib/UDP Send  InitFcn=|  FunctionName=sdspToNetwork  Parameters=localURL, localPortSource, localPort, remoteURL, remotePort, 8192, separateLengthPort, []  SFunctionDeploymentMode=off  EnableBusSupport=off  mask(UDP Send){remoteURL='192.168.140.159', remotePort=42784, localURL='0.0.0.0', localPortSource=Specify via dialog, localPort=42784, sampletime=-1, blockPlatform=Raspberry Pi, separateLengthPort=0}
      | realtime.internal.validateLinuxBlock(get_param(gcbh, 'blockPlatform'), gcbh);
      | realtime.internal.registerLinuxBlock(gcb);
      mask prompts: remoteURL "Remote IP address ('255.255.255.255' for broadcast):"; remotePort "Remote IP port:"; localURL "Local IP address:"; localPortSource "Local IP port source:"; localPort "Local IP port:"; blockPlatform "Block Platform"; separateLengthPort "Use a separate length port"
      mask help: Sends UDP packets to another UDP host on an Internet network. Set Remote IP address parameter to the IP address of the receiving UDP host. Set the Remote IP port parameter to the port number used by the receiving UDP host.
      mask Help: eval('realtime.helpView(get_param(gcb, ''blockPlatform''), [realtime.internal.getHelpLinkPrefix(gcb) ''libudpsend''])');
      mask TypeOptions localPortSource: Automatically determine | Specify via dialog
      mask Callback localPortSource:
      | mask_vis = get_param(gcbh, 'MaskVisibilities');
      | if strcmp(get_param(gcbh,'localPortSource'),'Specify via dialog')
      |     mask_vis{5} = 'on';
      | else
      |     mask_vis{5} = 'off';
      | end
      | set_param(gcbh, 'MaskVisibilities', mask_vis);
      | clear('mask_vis');
      mask Display:
      | %fprintf('UDP Send');
      | color('blue');
      | [data, map]=imread('ethernet2_bw.gif');pic=ind2rgb(data,map);image(pic,[0.32 0.25 0.40 0.45]);
      | platform = realtime.internal.getBlockDisplayText(gcb);
      | text(0.99, 0.9, platform, 'horizontalalignment', 'right');
  encode : MATLAB Function  Commented=on  TreatAsAtomicUnit=on
  wires:
  encode/1(serialized_data) -> ?
  data_out_C2C/1 -> Selector/1
  Data Type Conversion/1 -> UDP Send1/1
  Subsystem/1(Out1) -> Data Type Conversion/1
  Selector/1 -> Subsystem/1(In1)

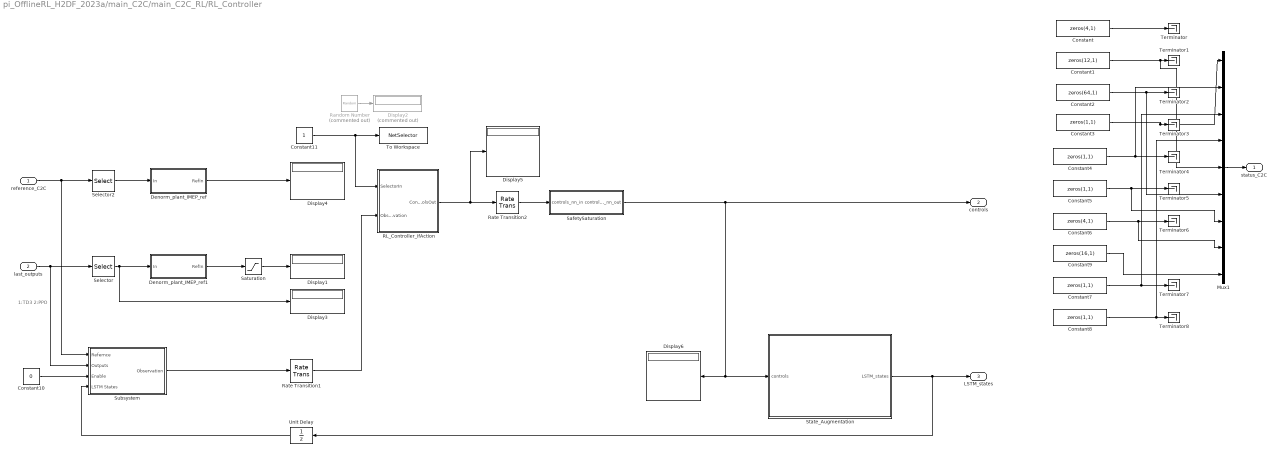
== system pi_OfflineRL_H2DF_2023a/main_C2C/main_C2C_RL/RL_Controller ==
  note: 1:TD3
      | 2:PPO
  reference_C2C : Inport
  last_outputs : Inport  Port=2
  Constant : Constant  Value=zeros(4,1)
  Constant1 : Constant  Value=zeros(12,1)
  Constant10 : Constant  Value=0
  Constant11 : Constant
  Constant2 : Constant  Value=zeros(64,1)
  Constant{3..5,7..8} (5 alike) : Constant  Value=zeros(1,1)
  Constant6 : Constant  Value=zeros(4,1)
  Constant9 : Constant  Value=zeros(16,1)
  Denorm_plant_IMEP_ref : Subsystem
  Denorm_plant_IMEP_ref1 : Subsystem
  Display{1,3..6} (5 alike) : Display
  Display2 : Display  Commented=on
  Mux1 : Mux  Inputs=9
  RL_Controller_ifAction : Subsystem  TreatAsAtomicUnit=on  PartitionName=part1
  Random Number : RandomNumber  Commented=on
  Rate Transition1 : RateTransition
  Rate Transition2 : RateTransition
  SafetySaturation : Subsystem
  Saturation : Saturate  UpperLimit=8.5e5  LowerLimit=3e5
  Selector : Selector  InputPortWidth=4  IndexOptions=Index vector (dialog)  Indices=[1]  OutputSizes=1
  Selector2 : Selector  IndexOptions=Index vector (dialog)  Indices=5  OutputSizes=1
  State_Augmentation : Subsystem
  Subsystem : Subsystem
  Terminator{,1..8} (9 alike) : Terminator
  To Workspace : ToWorkspace  VariableName=NetSelector  SampleTime=-1
      settings: Save2DSignal=2-D array (concatenate along first dimension)
  Unit Delay : UnitDelay  SampleTime=-1  HasFrameUpgradeWarning=on
  status_C2C : Outport
  controls : Outport  Port=2
  LSTM_states : Outport  Port=3
  wires:
  Constant4/1 -> Mux1/2, Terminator4/1
  Mux1/1 -> status_C2C/1
  Constant8/1 -> Terminator8/1, Mux1/4
  Constant7/1 -> Terminator7/1, Mux1/3
  Constant6/1 -> Terminator6/1, Mux1/8
  Constant5/1 -> Terminator5/1, Mux1/7
  Constant9/1 -> Mux1/9
  Constant3/1 -> Mux1/1, Terminator3/1
  Constant2/1 -> Terminator2/1, Mux1/6
  Constant1/1 -> Terminator1/1, Mux1/5
  Constant/1 -> Terminator/1
  Random Number/1 -> Display2/1
  Selector2/1 -> Denorm_plant_IMEP_ref/1(In)
  Saturation/1 -> Display1/1
  reference_C2C/1 -> Subsystem/1(Refernce), Selector2/1
  Selector/1 -> Denorm_plant_IMEP_ref1/1(In), Display3/1
  Denorm_plant_IMEP_ref/1(RefIn) -> Display4/1
  Denorm_plant_IMEP_ref1/1(RefIn) -> Saturation/1
  last_outputs/1 -> Selector/1, Subsystem/2(Outputs)
  RL_Controller_ifAction/1(ControlsOut) -> Display5/1, Rate Transition2/1
  Constant11/1 -> RL_Controller_ifAction/1(SelectorIn), To Workspace/1
  SafetySaturation/1(controls_nn_out) -> State_Augmentation/1(controls), Display6/1, controls/1
  Rate Transition2/1 -> SafetySaturation/1(controls_nn_in)
  Rate Transition1/1 -> RL_Controller_ifAction/2(Observation)
  State_Augmentation/1(LSTM_states) -> Unit Delay/1, LSTM_states/1
  Unit Delay/1 -> Subsystem/4(LSTM States)
  Subsystem/1(Observation) -> Rate Transition1/1
  Constant10/1 -> Subsystem/3(Enable)

== system pi_OfflineRL_H2DF_2023a/main_C2C/main_C2C_RL/post_processing ==
  reference : Inport
  controls : Inport  Port=2
  controller_status : Inport  Port=3
  last_outputs_MC : Inport  Port=4
  counter : Inport  Port=5
  LSTM_States : Inport  Port=6
  " denormalizing reference" : Subsystem
  Demux1 : Demux
  Demux2 : Demux
  Demux3 : Demux
  Display : Display  Commented=on
  Display1 : Display
  Mux{1,8..11} (5 alike) : Mux  Inputs=2
  Mux4 : Mux
  Mux5 : Mux  Inputs=6
  Mux6 : Mux
  Selector5 : Selector  IndexOptions=Index vector (dialog)  Indices=[(C2C_NMPC.Dims.n_controls + 1 ):(C2C_NMPC.Dims.n_cost - C2C_NMPC.Dims.n_controls)]  OutputSizes=1
  Subsystem : Subsystem  Commented=on
  Subsystem1 : Subsystem
  denormalizing physical controls and outputs : Subsystem
  data_C2C_out : Outport
  wires:
  Demux3/1 -> " denormalizing reference"/1(IMEP_norm)
  Demux3/2 -> " denormalizing reference"/2(NOX_norm)
  Demux3/4 -> " denormalizing reference"/4(MPRR_norm)
  Demux3/3 -> " denormalizing reference"/3(soot_norm)
  reference/1 -> Selector5/1
  Selector5/1 -> Demux3/1
  controls/1 -> Demux2/1
  Demux1/1 -> denormalizing physical controls and outputs/1(IMEP_norm)
  Demux1/2 -> denormalizing physical controls and outputs/2(NOX_norm)
  Demux1/3 -> denormalizing physical controls and outputs/3(soot_norm)
  Demux1/4 -> denormalizing physical controls and outputs/4(MPRR_norm)
  Demux2/1 -> denormalizing physical controls and outputs/5(DOI_main_norm)
  Demux2/2 -> denormalizing physical controls and outputs/6(SOI_pre_norm)
  Demux2/3 -> denormalizing physical controls and outputs/7(SOI_main_norm)
  denormalizing physical controls and outputs/5(DOI_main) -> Mux6/1
  denormalizing physical controls and outputs/6(SOI_pre) -> Mux6/2
  denormalizing physical controls and outputs/7(SOI_main) -> Mux6/3
  " denormalizing reference"/1(IMEP) -> Mux11/1
  " denormalizing reference"/2(NOX) -> Mux9/1
  " denormalizing reference"/3(soot) -> Mux8/1
  " denormalizing reference"/4(MPRR) -> Mux10/1
  controller_status/1 -> Mux5/4, Subsystem1/1(controller_ status), Subsystem/1(controller_ status)
  Mux5/1 -> data_C2C_out/1
  Mux8/1 -> Mux4/3
  Mux10/1 -> Mux4/4
  denormalizing physical controls and outputs/1(IMEP) -> Mux11/2
  denormalizing physical controls and outputs/2(NOX) -> Mux9/2
  denormalizing physical controls and outputs/3(soot) -> Mux8/2
  denormalizing physical controls and outputs/4(MPRR) -> Mux10/2
  Mux4/1 -> Mux5/2
  counter/1 -> Mux5/3
  Mux6/1 -> Display/1, Mux5/1
  Demux2/4 -> denormalizing physical controls and outputs/8(DOI_H2_norm)
  denormalizing physical controls and outputs/8(DOI_H2) -> Mux6/4
  Mux9/1 -> Mux4/2
  last_outputs_MC/1 -> Subsystem1/2(Last_Output_MC), Demux1/1
  Subsystem1/1(Out1) -> Mux5/6
  Mux11/1 -> Display1/1, Mux4/1
  LSTM_States/1 -> Mux1/2, Mux1/1
  Mux1/1 -> Mux5/5

== system pi_OfflineRL_H2DF_2023a/main_C2C/main_C2C_RL/pre_processing1 ==
  data_in_C2C : Inport
  Selector : Selector  IndexOptions=Index vector (dialog)  Indices=[6]  OutputSizes=1
  normalize_last_outputs_MC : Subsystem
  normalize_reference_C2C : Subsystem
  reference_C2C : Outport  VectorParamsAs1DForOutWhenUnconnected=off
  counter_C2C : Outport  Port=2  VectorParamsAs1DForOutWhenUnconnected=off
  last_outputs_MC : Outport  Port=3  VectorParamsAs1DForOutWhenUnconnected=off
  wires:
  normalize_reference_C2C/1(reference_C2C) -> reference_C2C/1
  data_in_C2C/1 -> Selector/1, normalize_last_outputs_MC/1(data_in), normalize_reference_C2C/1(data_in)
  normalize_last_outputs_MC/1(last_outputs_MC) -> last_outputs_MC/1
  Selector/1 -> counter_C2C/1

== system pi_OfflineRL_H2DF_2023a/main_C2C_RL/RL_Controller/Denorm_plant_IMEP_ref ==
  In : Inport
  Constant : Constant  Value=C2C_NMPC.Normalization.outputs.mean(1)
  Gain : Gain  Gain=C2C_NMPC.Normalization.outputs.std(1)
  Sum6 : Sum  Inputs=|++
  RefIn : Outport
  wires:
  In/1 -> Gain/1  "IMEP"
  Sum6/1 -> RefIn/1
  Gain/1 -> Sum6/1
  Constant/1 -> Sum6/2

== system pi_OfflineRL_H2DF_2023a/main_C2C_RL/RL_Controller/Denorm_plant_IMEP_ref1 ==
  In : Inport
  Constant : Constant  Value=C2C_NMPC.Normalization.outputs.mean(1)
  Gain : Gain  Gain=C2C_NMPC.Normalization.outputs.std(1)
  Sum6 : Sum  Inputs=|++
  RefIn : Outport
  wires:
  Constant/1 -> Sum6/2
  Gain/1 -> Sum6/1
  Sum6/1 -> RefIn/1
  In/1 -> Gain/1  "IMEP"

== system pi_OfflineRL_H2DF_2023a/main_C2C_RL/RL_Controller/RL_Controller_ifAction ==
  note: 1:TD3: trained without state feedback, no SOOT
      | 2:TD3: trained with state feedback, no SOOT
      | 3. TD3: random at this point
      | 4. TD3: TD3: trained with state feedback, no SOOT, good for higher loads
      | 5: 2:TD3: trained with state feedback, no SOOT
      | 6:2:TD3: trained withou state feedback, no SOOT
  SelectorIn : Inport
  reference_C2C : Inport  Port=2
  last_outputs : Inport  Port=3
  State_feedback : Inport  Port=4
  Enable : Inport  Port=5
  Display1 : Display
  Merge : Merge  Inputs=8
  Mux : Mux
  RL_Controller_PPO1 : Subsystem  VariantControl=fb_LSTM_321_syn
  RL_Controller_PPO2 : Subsystem  VariantControl=fb_LSTM_321_syn
  RL_Controller_PPO3 : Subsystem  VariantControl=fb_LSTM_321_syn
  RL_Controller_PPO4 : Subsystem  VariantControl=fb_LSTM_321_syn
  RL_Controller_PPO5 : Subsystem  VariantControl=fb_LSTM_321_syn
  RL_Controller_PPO6 : Subsystem  VariantControl=fb_LSTM_321_syn
  RL_Controller_PPO7 : Subsystem  VariantControl=fb_LSTM_321_syn
  RL_Controller_PPO8 : Subsystem  VariantControl=fb_LSTM_321_syn
  Switch Case : SwitchCase  CaseConditions={1,2,3,4,5,6,7,8}  ShowDefaultCase=off
  ControlsOut : Outport
  wires:
  SelectorIn/1 -> Switch Case/1
  Merge/1 -> ControlsOut/1, Display1/1
  RL_Controller_PPO5/1(Control_norm_NN_params) -> Merge/1
  RL_Controller_PPO6/1(Control_norm_NN_params) -> Merge/2
  Switch Case/1 -> RL_Controller_PPO5/Action
  Switch Case/2 -> RL_Controller_PPO6/Action
  Switch Case/3 -> RL_Controller_PPO1/Action
  RL_Controller_PPO1/1(Control_norm_NN_params) -> Merge/3
  reference_C2C/1 -> Mux/1
  last_outputs/1 -> Mux/2
  State_feedback/1 -> Mux/3
  Mux/1 -> RL_Controller_PPO5/1(In), RL_Controller_PPO6/1(In), RL_Controller_PPO1/1(In), RL_Controller_PPO8/1(In), RL_Controller_PPO7/1(In), RL_Controller_PPO4/1(In), RL_Controller_PPO3/1(In), RL_Controller_PPO2/1(In)
  Enable/1 -> Mux/4
  Switch Case/4 -> RL_Controller_PPO2/Action
  RL_Controller_PPO2/1(Control_norm_NN_params) -> Merge/4
  Switch Case/5 -> RL_Controller_PPO3/Action
  RL_Controller_PPO3/1(Control_norm_NN_params) -> Merge/5
  Switch Case/6 -> RL_Controller_PPO4/Action
  RL_Controller_PPO4/1(Control_norm_NN_params) -> Merge/6
  Switch Case/7 -> RL_Controller_PPO7/Action
  RL_Controller_PPO7/1(Control_norm_NN_params) -> Merge/7
  Switch Case/8 -> RL_Controller_PPO8/Action
  RL_Controller_PPO8/1(Control_norm_NN_params) -> Merge/8

== system pi_OfflineRL_H2DF_2023a/main_C2C_RL/RL_Controller/SafetySaturation ==
  controls_nn_in : Inport
  Saturation4 : Saturate  UpperLimit=UpperLimit  LowerLimit=LowerLimit
  controls_nn_out : Outport
  wires:
  controls_nn_in/1 -> Saturation4/1
  Saturation4/1 -> controls_nn_out/1
